simulink subsystem "gravitational_accelerations"  (R2023b)
settings: Solver=VariableStepAuto  StartTime=0.0  StopTime=10.0  RelTol=1e-3
libraries: dyn_lib x11
settings Model: Creator=brent  LastModifiedBy=brent

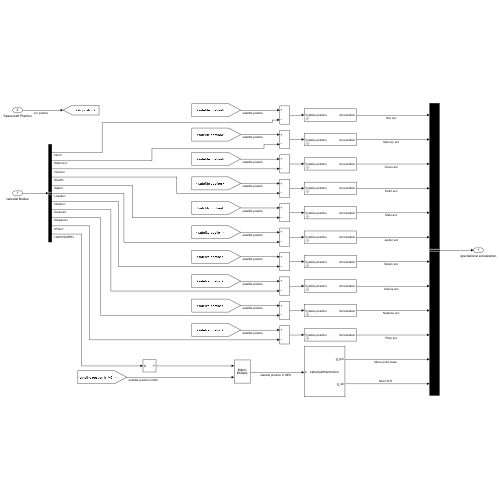
[thumbnail: Simulink's stored preview of the top-level diagram]
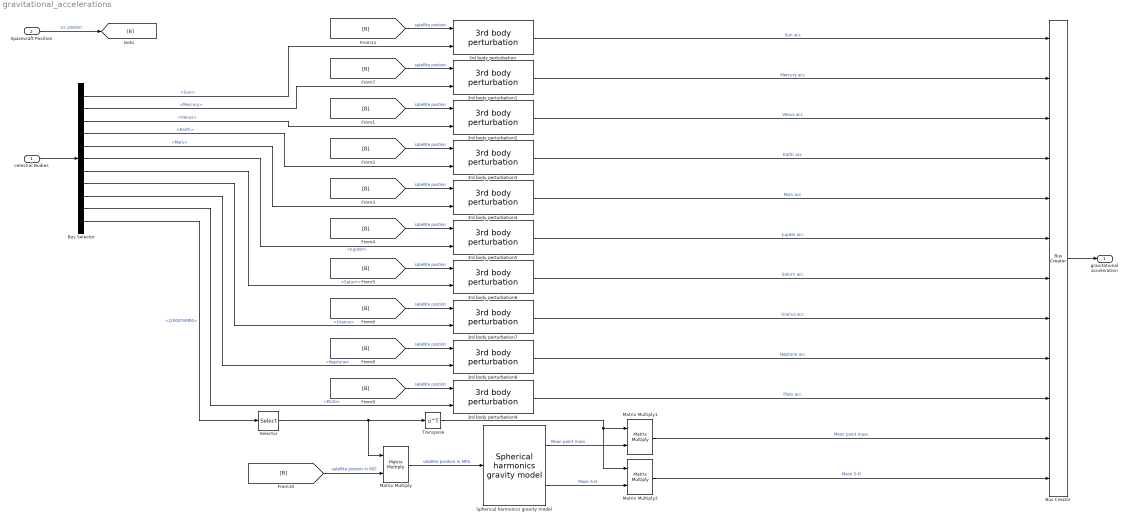
== system gravitational_accelerations ==
  celestial Bodies : Inport
  Spacecraft Position : Inport  Port=2
  3rd body perturbation : dyn_lib/3rd body perturbation  mu=Environment.Sun.mu.value
  3rd body perturbation1 : dyn_lib/3rd body perturbation  mu=Environment.Mercury.mu.value
  3rd body perturbation2 : dyn_lib/3rd body perturbation  mu=Environment.Venus.mu.value
  3rd body perturbation3 : dyn_lib/3rd body perturbation  mu=Environment.Earth.mu.value
  3rd body perturbation4 : dyn_lib/3rd body perturbation  mu=Environment.Mars.mu.value
  3rd body perturbation5 : dyn_lib/3rd body perturbation  mu=Environment.Jupiter.mu.value
  3rd body perturbation6 : dyn_lib/3rd body perturbation  mu=Environment.Saturn.mu.value
  3rd body perturbation7 : dyn_lib/3rd body perturbation  mu=Environment.Uranus.mu.value
  3rd body perturbation8 : dyn_lib/3rd body perturbation  mu=Environment.Neptune.mu.value
  3rd body perturbation9 : dyn_lib/3rd body perturbation  mu=Environment.Pluto.mu.value
  Bus Creator : BusCreator  Inputs=Sun acc,Mercury acc,Venus acc,Earth acc,Mars acc,Jupiter acc,Saturn acc,Uranus acc,Neptune acc,Pluto acc,Moon point mass,Moon S-H
  Bus Selector : BusSelector  OutputSignals=Sun,Mercury,Venus,Earth,Mars,Jupiter,Saturn,Uranus,Neptune,Pluto,J2000ToMPA
  Matrix Multiply : Product  Multiplication=Matrix(*)
  Matrix Multiply1 : Product  Multiplication=Matrix(*)
  Matrix Multiply2 : Product  Multiplication=Matrix(*)
  Selector : Selector  NumberOfDimensions=2  InputPortWidth=3  IndexOptions=Index vector (dialog),Index vector (dialog)  Indices=[1 2 3],[1 2 3]  OutputSizes=1,1
  Spherical harmonics gravity model : dyn_lib/Spherical harmonics gravity model  body_coeffs=Environment.Moon.SH  mu=Environment.Moon.mu.value  ref_radius=Environment.Moon.radius.value  nMax=Environment.Moon.SH.n.value  mMax=Environment.Moon.SH.m.value  SimulateUsing=Code generation
  Transpose : Math  Operator=transpose
  gravitational acceleration : Outport
  wires:
  Spacecraft Position/1 -> [B]  "s/c postion"
  celestial Bodies/1 -> Bus Selector/1
  Bus Selector/1 -> 3rd body perturbation/2  "<Sun>"
  Bus Selector/2 -> 3rd body perturbation1/2  "<Mercury>"
  Bus Creator/1 -> gravitational acceleration/1
  Spherical harmonics gravity model/1 -> Matrix Multiply1/2  "Moon point mass"
  Bus Selector/11 -> Selector/1  "<J2000ToMPA>"
  Selector/1 -> Transpose/1, Matrix Multiply/1
  [B] -> Matrix Multiply/2  "satellite postion in MCI"
  Matrix Multiply/1 -> Spherical harmonics gravity model/1  "satellite position in MPA"
  Matrix Multiply1/1 -> Bus Creator/11  "Moon point mass"
  Transpose/1 -> Matrix Multiply1/1, Matrix Multiply2/1
  Spherical harmonics gravity model/2 -> Matrix Multiply2/2  "Moon S-H"
  Matrix Multiply2/1 -> Bus Creator/12  "Moon S-H"
  3rd body perturbation/1 -> Bus Creator/1  "Sun acc"
  3rd body perturbation1/1 -> Bus Creator/2  "Mercury acc"
  3rd body perturbation2/1 -> Bus Creator/3  "Venus acc"
  [B] -> 3rd body perturbation2/1  "satellite postion"
  Bus Selector/3 -> 3rd body perturbation2/2  "<Venus>"
  Bus Selector/4 -> 3rd body perturbation3/2  "<Earth>"
  3rd body perturbation3/1 -> Bus Creator/4  "Earth acc"
  Bus Selector/5 -> 3rd body perturbation4/2  "<Mars>"
  3rd body perturbation4/1 -> Bus Creator/5  "Mars acc"
  Bus Selector/6 -> 3rd body perturbation5/2  "<Jupiter>"
  [B] -> 3rd body perturbation5/1  "satellite postion"
  3rd body perturbation5/1 -> Bus Creator/6  "Jupiter acc"
  Bus Selector/7 -> 3rd body perturbation6/2  "<Saturn>"
  3rd body perturbation6/1 -> Bus Creator/7  "Saturn acc"
  Bus Selector/8 -> 3rd body perturbation7/2  "<Uranus>"
  3rd body perturbation7/1 -> Bus Creator/8  "Uranus acc"
  Bus Selector/9 -> 3rd body perturbation8/2  "<Neptune>"
  [B] -> 3rd body perturbation8/1  "satellite postion"
  3rd body perturbation8/1 -> Bus Creator/9  "Neptune acc"
  Bus Selector/10 -> 3rd body perturbation9/2  "<Pluto>"
  [B] -> 3rd body perturbation9/1  "satellite postion"
  3rd body perturbation9/1 -> Bus Creator/10  "Pluto acc"
  [B] -> 3rd body perturbation/1  "satellite postion"
  [B] -> 3rd body perturbation1/1  "satellite postion"
  [B] -> 3rd body perturbation3/1  "satellite postion"
  [B] -> 3rd body perturbation4/1  "satellite postion"
  [B] -> 3rd body perturbation6/1  "satellite postion"
  [B] -> 3rd body perturbation7/1  "satellite postion"
